simulink model "sm_boom_lift_crawler_abstract_flex_boom"  (R2026a)
settings: Solver=ode23t  StopTime=operator_seq.StopTime  FixedStep=2e-2  MaxStep=2  AbsTol=1e-3
PreLoadFcn:
  | sm_boom_lift_crawler_settest('full test')
StartFcn:
  | tic;
StopFcn:
  | Elapsed_Sim_Time = toc;
  | %disp(['Elapsed Sim Time = ' num2str(Elapsed_Sim_Time)]);
undefined symbols (not defined in the file or in its folder): b, BasketR, Boom, Chassis, Extend, FL, FR, Jib, LevelM, LevelS, Lift, operator_seq, OutFL, OutFR, OutRL, OutRR, RL, RR, Tilt, TrackL, TrackR, Turret, X, Y, Z
libraries: sm_lib x67, sm_boom_lift_crawler_lib x22, nesl_utility x15, sm_boom_lift_crawler_lib_boom x5, sm_boom_lift_crawler_lib_control x1, sm_boom_lift_crawler_lib_chassis x1
(part 5 of 5)

== system sm_boom_lift_crawler_abstract_flex_boom/Lift/Boom/Arms/Subsystem2/Transform Flex Beam/Align Joint ==
  Rigid Transform2 : sm_lib/Frames and Transforms/Rigid Transform  RotationMethod=StandardAxis  FollAlignAxisA=+X  BaseAlignAxisA=+Y  FollAlignAxisB=+Y  BaseAlignAxisB=+Z  RotationStandardAxis=+Y  RotationAngle=90  RotationAngleUnits=deg  RotationArbitraryAxis=[0 0 1]  RotationSequenceAxes=FollowerAxes  RotationSequence=XYX  RotationSequenceAngles=[0 0 0]  RotationSequenceAnglesUnits=deg  RotationMatrix=[1 0 0; 0 1 0; 0 0 1]  Quaternion=[1 0 0 0]  TranslationMethod=None  TranslationCartesianOffset=[0 0 0]  TranslationCartesianOffsetUnits=m  TranslationStandardAxis=+Z  TranslationStandardOffset=0  TranslationStandardOffsetUnits=m  TranslationROffset=0  TranslationROffsetUnits=m  TranslationThetaOffset=0  TranslationThetaOffsetUnits=deg  TranslationZOffset=0  TranslationZOffsetUnits=m
  Rigid Transform3 : sm_lib/Frames and Transforms/Rigid Transform  RotationMethod=StandardAxis  FollAlignAxisA=+X  BaseAlignAxisA=+Y  FollAlignAxisB=+Y  BaseAlignAxisB=+Z  RotationStandardAxis=+Z  RotationAngle=-90  RotationAngleUnits=deg  RotationArbitraryAxis=[0 0 1]  RotationSequenceAxes=FollowerAxes  RotationSequence=XYX  RotationSequenceAngles=[0 0 0]  RotationSequenceAnglesUnits=deg  RotationMatrix=[1 0 0; 0 1 0; 0 0 1]  Quaternion=[1 0 0 0]  TranslationMethod=None  TranslationCartesianOffset=[0 0 0]  TranslationCartesianOffsetUnits=m  TranslationStandardAxis=+Z  TranslationStandardOffset=0  TranslationStandardOffsetUnits=m  TranslationROffset=0  TranslationROffsetUnits=m  TranslationThetaOffset=0  TranslationThetaOffsetUnits=deg  TranslationZOffset=0  TranslationZOffsetUnits=m
  B : PMIOPort  Side=Left
  F : PMIOPort  Port=2  Side=Right
  connections:
  Rigid Transform3/RConn1 -- Rigid Transform2/LConn1
  Rigid Transform3/LConn1 -- B/RConn1
  Rigid Transform2/RConn1 -- F/RConn1

== system sm_boom_lift_crawler_abstract_flex_boom/Lift/Boom/Arms/Telescoping Boom Flex/Classical/Base Beam ==
  Base Beam : sm_lib/Body Elements/Flexible Bodies/Beams/Flexible Rectangular Beam  SectionType=Hollow  Width=base_w  WidthUnits=ft  Height=base_h  HeightUnits=ft  Thickness=base_t  ThicknessUnits=ft  Length=base_l-overlap_l  LengthUnits=ft  StiffnessAndInertiaType=CalculateFromGeometry  Density=base_rho  DensityUnits=kg/m^3  ModuliType=YoungsPoissons  YoungsModulus=base_E  YoungsModulusUnits=GPa  PoissonsRatio=base_v  ShearModulus=26  ShearModulusUnits=GPa  GeometricCentroid=[0 0]  GeometricCentroidUnits=m  BendingCentroid=[0 0]  BendingCentroidUnits=m  ShearCenter=[0 0]  ShearCenterUnits=m  AxialRigidity=1  AxialRigidityUnits=Pa*m^2  FlexuralRigidity=[1 1]  FlexuralRigidityUnits=Pa*m^4  CrossFlexuralRigidity=0  CrossFlexuralRigidityUnits=Pa*m^4  TorsionalRigidity=1  TorsionalRigidityUnits=Pa*m^4  CenterOfMass=[0 0]  CenterOfMassUnits=m  MassPerUnitLength=1  MassPerUnitLengthUnits=kg/m  MassMomentOfInertiaDensity=[1 1]  MassMomentOfInertiaDensityUnits=kg*m  MassProductOfInertiaDensity=0  MassProductOfInertiaDensityUnits=kg*m  DampingType=Proportional  ProportionalDampingAlpha=0  ProportionalDampingAlphaUnits=1/s  ProportionalDampingBeta=0.001  ProportionalDampingBetaUnits=s  UniformModalDampingRatio=0.01  NumElements=1  ReferenceConditionsType=LinearizedMeanAxes  DoExposeReferenceFrame=off  ReductionType=None  NumRetainedModes=1  GraphicType=FromGeometry  GraphicVisPropType=AdvancedVisualProperties  GraphicDiffuseColor=base_clr_d  GraphicOpacity=base_opc  GraphicSpecularColor=base_clr_s  GraphicAmbientColor=base_clr_a  GraphicEmissiveColor=base_clr_e  GraphicShininess=base_clr_h  DoExposeZminFrame=on  DoExposeZmaxFrame=on  SerializedFrames=<Frames/>
  Overlap Base Mid : sm_boom_lift_crawler_lib/Beam Rigid Segment  beam_h=base_h  beam_w=base_w  beam_t=base_t  beam_l=overlap_l  beam_rho=base_rho  clr_d=base_clr_d  clr_s=base_clr_s  clr_a=base_clr_a  clr_e=base_clr_e  clr_h=base_clr_h  opc=base_opc
  B : PMIOPort  Side=Left
  F : PMIOPort  Port=2  Side=Right
  connections:
  Overlap Base Mid/LConn1 -- Base Beam/RConn1
  B/RConn1 -- Base Beam/LConn1
  Overlap Base Mid/RConn1 -- F/RConn1

== system sm_boom_lift_crawler_abstract_flex_boom/Lift/Boom/Arms/Telescoping Boom Flex/Classical/Fly Beam ==
  Fly Beam : sm_lib/Body Elements/Flexible Bodies/Beams/Flexible Rectangular Beam  SectionType=Hollow  Width=fly_w  WidthUnits=ft  Height=fly_h  HeightUnits=ft  Thickness=fly_t  ThicknessUnits=ft  Length=fly_l-overlap_l  LengthUnits=ft  StiffnessAndInertiaType=CalculateFromGeometry  Density=fly_rho  DensityUnits=kg/m^3  ModuliType=YoungsPoissons  YoungsModulus=fly_E  YoungsModulusUnits=GPa  PoissonsRatio=fly_v  ShearModulus=26  ShearModulusUnits=GPa  GeometricCentroid=[0 0]  GeometricCentroidUnits=m  BendingCentroid=[0 0]  BendingCentroidUnits=m  ShearCenter=[0 0]  ShearCenterUnits=m  AxialRigidity=1  AxialRigidityUnits=Pa*m^2  FlexuralRigidity=[1 1]  FlexuralRigidityUnits=Pa*m^4  CrossFlexuralRigidity=0  CrossFlexuralRigidityUnits=Pa*m^4  TorsionalRigidity=1  TorsionalRigidityUnits=Pa*m^4  CenterOfMass=[0 0]  CenterOfMassUnits=m  MassPerUnitLength=1  MassPerUnitLengthUnits=kg/m  MassMomentOfInertiaDensity=[1 1]  MassMomentOfInertiaDensityUnits=kg*m  MassProductOfInertiaDensity=0  MassProductOfInertiaDensityUnits=kg*m  DampingType=Proportional  ProportionalDampingAlpha=0  ProportionalDampingAlphaUnits=1/s  ProportionalDampingBeta=0.001  ProportionalDampingBetaUnits=s  UniformModalDampingRatio=0.01  NumElements=1  ReferenceConditionsType=LinearizedMeanAxes  DoExposeReferenceFrame=off  ReductionType=None  NumRetainedModes=1  GraphicType=FromGeometry  GraphicVisPropType=AdvancedVisualProperties  GraphicDiffuseColor=fly_clr_d  GraphicOpacity=fly_opc  GraphicSpecularColor=fly_clr_s  GraphicAmbientColor=fly_clr_a  GraphicEmissiveColor=fly_clr_e  GraphicShininess=fly_clr_h  DoExposeZminFrame=on  DoExposeZmaxFrame=on  SerializedFrames=<Frames/>
  Overlap Fly Mid : sm_boom_lift_crawler_lib/Beam Rigid Segment  beam_h=fly_h  beam_w=fly_w  beam_t=fly_t  beam_l=fly_l  beam_rho=fly_rho  clr_d=fly_clr_d  clr_s=fly_clr_s  clr_a=fly_clr_a  clr_e=fly_clr_e  clr_h=fly_clr_h  opc=fly_opc
  Rigid Transform3 : sm_lib/Frames and Transforms/Rigid Transform  RotationMethod=None  FollAlignAxisA=+X  BaseAlignAxisA=+Y  FollAlignAxisB=+Y  BaseAlignAxisB=+Z  RotationStandardAxis=+Z  RotationAngle=0.0  RotationAngleUnits=deg  RotationArbitraryAxis=[0 0 1]  RotationSequenceAxes=FollowerAxes  RotationSequence=XYX  RotationSequenceAngles=[0 0 0]  RotationSequenceAnglesUnits=deg  RotationMatrix=[1 0 0; 0 1 0; 0 0 1]  Quaternion=[1 0 0 0]  TranslationMethod=StandardAxis  TranslationCartesianOffset=[0 0 0]  TranslationCartesianOffsetUnits=ft  TranslationStandardAxis=+Z  TranslationStandardOffset=-overlap_l  TranslationStandardOffsetUnits=ft  TranslationROffset=0  TranslationROffsetUnits=m  TranslationThetaOffset=0  TranslationThetaOffsetUnits=deg  TranslationZOffset=0  TranslationZOffsetUnits=m
  B : PMIOPort  Side=Left
  F : PMIOPort  Port=2  Side=Right
  connections:
  Overlap Fly Mid/RConn1 -- Fly Beam/LConn1
  Rigid Transform3/LConn1 -- B/RConn1
  Overlap Fly Mid/LConn1 -- Rigid Transform3/RConn1
  Fly Beam/RConn1 -- F/RConn1

== system sm_boom_lift_crawler_abstract_flex_boom/Lift/Boom/Arms/Telescoping Boom Flex/Classical/Mid Beam ==
  "Middle Beam " : sm_lib/Body Elements/Flexible Bodies/Beams/Flexible Rectangular Beam  SectionType=Hollow  Width=mid_w  WidthUnits=ft  Height=mid_h  HeightUnits=ft  Thickness=mid_t  ThicknessUnits=ft  Length=mid_l-2*overlap_l  LengthUnits=ft  StiffnessAndInertiaType=CalculateFromGeometry  Density=mid_rho  DensityUnits=kg/m^3  ModuliType=YoungsPoissons  YoungsModulus=mid_E  YoungsModulusUnits=GPa  PoissonsRatio=mid_v  ShearModulus=26  ShearModulusUnits=GPa  GeometricCentroid=[0 0]  GeometricCentroidUnits=m  BendingCentroid=[0 0]  BendingCentroidUnits=m  ShearCenter=[0 0]  ShearCenterUnits=m  AxialRigidity=1  AxialRigidityUnits=Pa*m^2  FlexuralRigidity=[1 1]  FlexuralRigidityUnits=Pa*m^4  CrossFlexuralRigidity=0  CrossFlexuralRigidityUnits=Pa*m^4  TorsionalRigidity=1  TorsionalRigidityUnits=Pa*m^4  CenterOfMass=[0 0]  CenterOfMassUnits=m  MassPerUnitLength=1  MassPerUnitLengthUnits=kg/m  MassMomentOfInertiaDensity=[1 1]  MassMomentOfInertiaDensityUnits=kg*m  MassProductOfInertiaDensity=0  MassProductOfInertiaDensityUnits=kg*m  DampingType=Proportional  ProportionalDampingAlpha=0  ProportionalDampingAlphaUnits=1/s  ProportionalDampingBeta=0.001  ProportionalDampingBetaUnits=s  UniformModalDampingRatio=0.01  NumElements=1  ReferenceConditionsType=LinearizedMeanAxes  DoExposeReferenceFrame=off  ReductionType=None  NumRetainedModes=1  GraphicType=FromGeometry  GraphicVisPropType=AdvancedVisualProperties  GraphicDiffuseColor=mid_clr_d  GraphicOpacity=mid_opc  GraphicSpecularColor=mid_clr_s  GraphicAmbientColor=mid_clr_a  GraphicEmissiveColor=mid_clr_e  GraphicShininess=mid_clr_h  DoExposeZminFrame=on  DoExposeZmaxFrame=on  SerializedFrames=<Frames/>
  Overlap Mid Base : sm_boom_lift_crawler_lib/Beam Rigid Segment  beam_h=mid_h  beam_w=mid_w  beam_t=mid_t  beam_l=mid_l  beam_rho=mid_rho  clr_d=mid_clr_d  clr_s=mid_clr_s  clr_a=mid_clr_a  clr_e=mid_clr_e  clr_h=mid_clr_h  opc=mid_opc
  Overlap Mid Fly : sm_boom_lift_crawler_lib/Beam Rigid Segment  beam_h=mid_h  beam_w=mid_w  beam_t=mid_t  beam_l=mid_l  beam_rho=mid_rho  clr_d=mid_clr_d  clr_s=mid_clr_s  clr_a=mid_clr_a  clr_e=mid_clr_e  clr_h=mid_clr_h  opc=mid_opc
  Transform Overlap B : sm_lib/Frames and Transforms/Rigid Transform  RotationMethod=None  FollAlignAxisA=+X  BaseAlignAxisA=+Y  FollAlignAxisB=+Y  BaseAlignAxisB=+Z  RotationStandardAxis=+Z  RotationAngle=0.0  RotationAngleUnits=deg  RotationArbitraryAxis=[0 0 1]  RotationSequenceAxes=FollowerAxes  RotationSequence=XYX  RotationSequenceAngles=[0 0 0]  RotationSequenceAnglesUnits=deg  RotationMatrix=[1 0 0; 0 1 0; 0 0 1]  Quaternion=[1 0 0 0]  TranslationMethod=StandardAxis  TranslationCartesianOffset=[0 0 0]  TranslationCartesianOffsetUnits=ft  TranslationStandardAxis=+Z  TranslationStandardOffset=-overlap_l  TranslationStandardOffsetUnits=ft  TranslationROffset=0  TranslationROffsetUnits=m  TranslationThetaOffset=0  TranslationThetaOffsetUnits=deg  TranslationZOffset=0  TranslationZOffsetUnits=m
  B : PMIOPort  Side=Left
  F : PMIOPort  Port=2  Side=Right
  connections:
  Overlap Mid Fly/RConn1 -- F/RConn1
  "Middle Beam "/RConn1 -- Overlap Mid Fly/LConn1
  Overlap Mid Base/LConn1 -- Transform Overlap B/RConn1
  Transform Overlap B/LConn1 -- B/RConn1
  "Middle Beam "/LConn1 -- Overlap Mid Base/RConn1

== system sm_boom_lift_crawler_abstract_flex_boom/Lift/Boom/Arms/Telescoping Boom Flex/ROM/Base Beam ==
  Overlap Base Mid : sm_boom_lift_crawler_lib/Beam Rigid Segment  beam_h=base_h  beam_w=base_w  beam_t=base_t  beam_l=overlap_l  beam_rho=base_rho  clr_d=base_clr_d  clr_s=base_clr_s  clr_a=base_clr_a  clr_e=base_clr_e  clr_h=base_clr_h  opc=base_opc
  Reduced Order Flexible Solid : sm_lib/Body Elements/Flexible Bodies/Reduced Order Flexible Solid  UnitSystemType=SI  LengthUnit=m  MassUnit=kg  TimeUnit=s  NumberOfInterfaceFrames=2  InterfaceFrameOrigins=origins_b20  InterfaceFrameOrientations=repmat([1 0 0 0],2,1)  StiffnessMatrix=ROM_b20.K  MassMatrix=ROM_b20.M  DampingType=DampingMatrix  ProportionalDampingAlpha=0  ProportionalDampingBeta=0.001  UniformModalDampingRatio=0.01  DampingMatrix=ROM_b20.C  ReferenceConditionsType=LinearizedMeanAxes  DoExposeReferenceFrame=off  ReductionType=None  NumRetainedModes=1  GraphicType=PartitionedGeometry  GeomFileName=Base_20.STL  GeomUnitType=FromUnitSystem  VisRecursionLimit=3  GraphicVertexCoordinates=[]  GraphicFacetVertexIndices=[]  GraphicReconstructionMatrix=[]  GraphicVisPropType=AdvancedVisualProperties  GraphicDiffuseColor=base_clr_d  GraphicOpacity=1.0  GraphicSpecularColor=base_clr_s  GraphicAmbientColor=base_clr_a  GraphicEmissiveColor=base_clr_e  GraphicShininess=base_clr_h  SenseReducedOrderDOFPosition=off  SenseReducedOrderDOFVelocity=off  SenseReducedOrderDOFAcceleration=off
  B : PMIOPort  Side=Left
  F : PMIOPort  Port=2  Side=Right
  connections:
  Overlap Base Mid/RConn1 -- F/RConn1
  Reduced Order Flexible Solid/LConn1 -- B/RConn1
  Reduced Order Flexible Solid/RConn1 -- Overlap Base Mid/LConn1

== system sm_boom_lift_crawler_abstract_flex_boom/Lift/Boom/Arms/Telescoping Boom Flex/ROM/Fly Beam ==
  Overlap Fly Mid : sm_boom_lift_crawler_lib/Beam Rigid Segment  beam_h=fly_h  beam_w=fly_w  beam_t=fly_t  beam_l=fly_l  beam_rho=fly_rho  clr_d=fly_clr_d  clr_s=fly_clr_s  clr_a=fly_clr_a  clr_e=fly_clr_e  clr_h=fly_clr_h  opc=fly_opc
  Reduced Order Flexible Solid : sm_lib/Body Elements/Flexible Bodies/Reduced Order Flexible Solid  UnitSystemType=SI  LengthUnit=m  MassUnit=kg  TimeUnit=s  NumberOfInterfaceFrames=2  InterfaceFrameOrigins=origins_f20  InterfaceFrameOrientations=repmat([1 0 0 0],2,1)  StiffnessMatrix=ROM_f20.K  MassMatrix=ROM_f20.M  DampingType=DampingMatrix  ProportionalDampingAlpha=0  ProportionalDampingBeta=0.001  UniformModalDampingRatio=0.01  DampingMatrix=ROM_f20.C  ReferenceConditionsType=LinearizedMeanAxes  DoExposeReferenceFrame=off  ReductionType=None  NumRetainedModes=1  GraphicType=PartitionedGeometry  GeomFileName=Fly_20.STL  GeomUnitType=FromUnitSystem  VisRecursionLimit=3  GraphicVertexCoordinates=[]  GraphicFacetVertexIndices=[]  GraphicReconstructionMatrix=[]  GraphicVisPropType=AdvancedVisualProperties  GraphicDiffuseColor=fly_clr_d  GraphicOpacity=1.0  GraphicSpecularColor=fly_clr_s  GraphicAmbientColor=fly_clr_a  GraphicEmissiveColor=fly_clr_e  GraphicShininess=fly_clr_h  SenseReducedOrderDOFPosition=off  SenseReducedOrderDOFVelocity=off  SenseReducedOrderDOFAcceleration=off
  Rigid Transform3 : sm_lib/Frames and Transforms/Rigid Transform  RotationMethod=None  FollAlignAxisA=+X  BaseAlignAxisA=+Y  FollAlignAxisB=+Y  BaseAlignAxisB=+Z  RotationStandardAxis=+Z  RotationAngle=0.0  RotationAngleUnits=deg  RotationArbitraryAxis=[0 0 1]  RotationSequenceAxes=FollowerAxes  RotationSequence=XYX  RotationSequenceAngles=[0 0 0]  RotationSequenceAnglesUnits=deg  RotationMatrix=[1 0 0; 0 1 0; 0 0 1]  Quaternion=[1 0 0 0]  TranslationMethod=StandardAxis  TranslationCartesianOffset=[0 0 0]  TranslationCartesianOffsetUnits=ft  TranslationStandardAxis=+Z  TranslationStandardOffset=-overlap_l  TranslationStandardOffsetUnits=ft  TranslationROffset=0  TranslationROffsetUnits=m  TranslationThetaOffset=0  TranslationThetaOffsetUnits=deg  TranslationZOffset=0  TranslationZOffsetUnits=m
  B : PMIOPort  Side=Left
  F : PMIOPort  Port=2  Side=Right
  connections:
  Reduced Order Flexible Solid/RConn1 -- F/RConn1
  Overlap Fly Mid/LConn1 -- Rigid Transform3/RConn1
  Rigid Transform3/LConn1 -- B/RConn1
  Reduced Order Flexible Solid/LConn1 -- Overlap Fly Mid/RConn1

== system sm_boom_lift_crawler_abstract_flex_boom/Lift/Boom/Arms/Telescoping Boom Flex/ROM/Mid Beam ==
  Overlap Mid Base : sm_boom_lift_crawler_lib/Beam Rigid Segment  beam_h=mid_h  beam_w=mid_w  beam_t=mid_t  beam_l=mid_l  beam_rho=mid_rho  clr_d=mid_clr_d  clr_s=mid_clr_s  clr_a=mid_clr_a  clr_e=mid_clr_e  clr_h=mid_clr_h  opc=mid_opc
  Overlap Mid Fly : sm_boom_lift_crawler_lib/Beam Rigid Segment  beam_h=mid_h  beam_w=mid_w  beam_t=mid_t  beam_l=mid_l  beam_rho=mid_rho  clr_d=mid_clr_d  clr_s=mid_clr_s  clr_a=mid_clr_a  clr_e=mid_clr_e  clr_h=mid_clr_h  opc=mid_opc
  Reduced Order Flexible Solid : sm_lib/Body Elements/Flexible Bodies/Reduced Order Flexible Solid  UnitSystemType=SI  LengthUnit=m  MassUnit=kg  TimeUnit=s  NumberOfInterfaceFrames=2  InterfaceFrameOrigins=origins_m20  InterfaceFrameOrientations=repmat([1 0 0 0],2,1)  StiffnessMatrix=ROM_m20.K  MassMatrix=ROM_m20.M  DampingType=DampingMatrix  ProportionalDampingAlpha=0  ProportionalDampingBeta=0.001  UniformModalDampingRatio=0.01  DampingMatrix=ROM_m20.C  ReferenceConditionsType=LinearizedMeanAxes  DoExposeReferenceFrame=off  ReductionType=None  NumRetainedModes=1  GraphicType=PartitionedGeometry  GeomFileName=Mid_20.STL  GeomUnitType=FromUnitSystem  VisRecursionLimit=3  GraphicVertexCoordinates=[]  GraphicFacetVertexIndices=[]  GraphicReconstructionMatrix=[]  GraphicVisPropType=AdvancedVisualProperties  GraphicDiffuseColor=mid_clr_d  GraphicOpacity=1.0  GraphicSpecularColor=mid_clr_s  GraphicAmbientColor=mid_clr_a  GraphicEmissiveColor=mid_clr_e  GraphicShininess=mid_clr_h  SenseReducedOrderDOFPosition=off  SenseReducedOrderDOFVelocity=off  SenseReducedOrderDOFAcceleration=off
  Rigid Transform2 : sm_lib/Frames and Transforms/Rigid Transform  RotationMethod=None  FollAlignAxisA=+X  BaseAlignAxisA=+Y  FollAlignAxisB=+Y  BaseAlignAxisB=+Z  RotationStandardAxis=+Z  RotationAngle=0.0  RotationAngleUnits=deg  RotationArbitraryAxis=[0 0 1]  RotationSequenceAxes=FollowerAxes  RotationSequence=XYX  RotationSequenceAngles=[0 0 0]  RotationSequenceAnglesUnits=deg  RotationMatrix=[1 0 0; 0 1 0; 0 0 1]  Quaternion=[1 0 0 0]  TranslationMethod=StandardAxis  TranslationCartesianOffset=[0 0 0]  TranslationCartesianOffsetUnits=ft  TranslationStandardAxis=+Z  TranslationStandardOffset=-overlap_l  TranslationStandardOffsetUnits=ft  TranslationROffset=0  TranslationROffsetUnits=m  TranslationThetaOffset=0  TranslationThetaOffsetUnits=deg  TranslationZOffset=0  TranslationZOffsetUnits=m
  B : PMIOPort  Side=Left
  F : PMIOPort  Port=2  Side=Right
  connections:
  Reduced Order Flexible Solid/LConn1 -- Overlap Mid Base/RConn1
  Rigid Transform2/LConn1 -- B/RConn1
  Overlap Mid Base/LConn1 -- Rigid Transform2/RConn1
  Reduced Order Flexible Solid/RConn1 -- Overlap Mid Fly/LConn1
  Overlap Mid Fly/RConn1 -- F/RConn1
